simulink model "Aerosonde_NON_linear"  (R2023b)
settings: Solver=VariableStepAuto  StartTime=0.0  StopTime=30  RelTol=1e-3
InitFcn:
  | X0 = [0; 2; -0.25; 0.01; 0; 0; 0; 0; 0; 0; 0; 0]
values from neighbouring files (symbols this model uses):
  kd_pitch = (2*zita_pitch * wn_pitch -a_teta1)/a_teta3    [aerosonde_NON_linear_model.m]
  kd_roll = (2*zita_phi*wn_roll-a_phi1)/a_phi2    [aerosonde_NON_linear_model.m]
  ki_beta = wn_beta^2/a_beta2    (= -1631.35406636)    [aerosonde_NON_linear_model.m]
  ki_course = wn_course^2*Vg/gravity    [aerosonde_NON_linear_model.m]
  ki_h = wn_h^2/(Va*K_pitch_DC)    [aerosonde_NON_linear_model.m]
  ki_v = wn_V^2 / a_v2    (= 0.410281846391)    [aerosonde_NON_linear_model.m]
  ki_v2 = -wn_V2^2/gravity/K_pitch_DC    [aerosonde_NON_linear_model.m]
  kp_beta = delta_r_max/e_beta_max    (= -61)    [aerosonde_NON_linear_model.m]
  kp_course = 2*zita_course*wn_course*Vg/gravity    [aerosonde_NON_linear_model.m]
  kp_h = 2*zita_h*wn_h/(Va*K_pitch_DC)    [aerosonde_NON_linear_model.m]
  kp_pitch = delta_e_max / e_teta_max * sign(a_teta3)    [aerosonde_NON_linear_model.m]
  kp_roll = delta_a_max/e_phi_max    (= 1.04)    [aerosonde_NON_linear_model.m]
  kp_v = (2*zita_V*wn_V-a_v1)/a_v2    (= 0.315424848104)    [aerosonde_NON_linear_model.m]
  kp_v2 = -(a_v1 - 2*zita_V2 * wn_V2)/gravity/K_pitch_DC    [aerosonde_NON_linear_model.m]
  Lu = 300    [aerosonde_NON_linear_model.m]
  Lv = Lu    (= 300)    [aerosonde_NON_linear_model.m]
  Lw = 100    [aerosonde_NON_linear_model.m]
  sigma_u = 2.12    [aerosonde_NON_linear_model.m]
  sigma_v = sigma_u    (= 2.12)    [aerosonde_NON_linear_model.m]
  sigma_w = 1.4    [aerosonde_NON_linear_model.m]
  Va = [0.01 0.01 0.0102487877003 0.0114927261887 0.0177124182161 0.0248890223027 0.0320656246486 0.0395378524425 0.0423652294331 0.0451926059638 0.0466645323698 0.0481364586384 ... (831 elements, 831x1)]    [Vae1.mat]    (also in Vae2.mat = [0.01 0.01 0.0102487877003 0.0114927261887 0.0177124182161 0; Vae3.mat = [0.01 0.01 0.0102487877003 0.0114927261887 0.0177124182161 0; Vze2.mat = [0.01 0.01 0.0102487877003 0.0114927261887 0.0177124182161 0; Vze3.mat = [0.01 0.01 0.0102487877003 0.0114927261887 0.0177124182161 0)
libraries: simulink_extras x15, slpidlib x6, simulink x2, sim3dlib x1, uavsim3dlib x1
settings Model: Creator=Marco  LastModifiedBy=sasi
settings SolverCC: ZeroCrossAlgorithm=Adaptive
settings DebuggingCC: IgnoredZcDiagnostic=none  UnconnectedInputMsg=warning  UnconnectedOutputMsg=warning  UnconnectedLineMsg=warning
settings ModelReferenceCC: EnableRefExpFcnMdlSchedulingChecks=on
settings RTWCC: DLArmComputeVersion=19.05

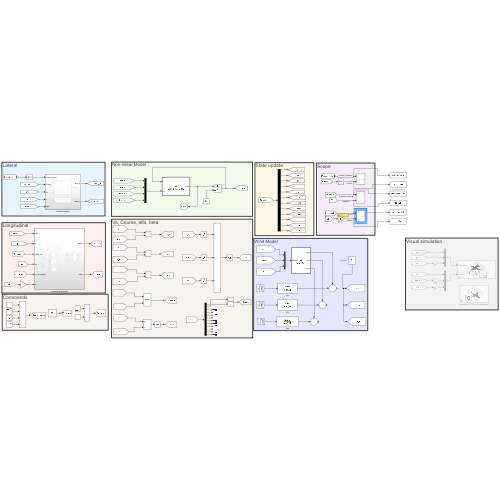
[thumbnail: Simulink's stored preview of the top-level diagram]
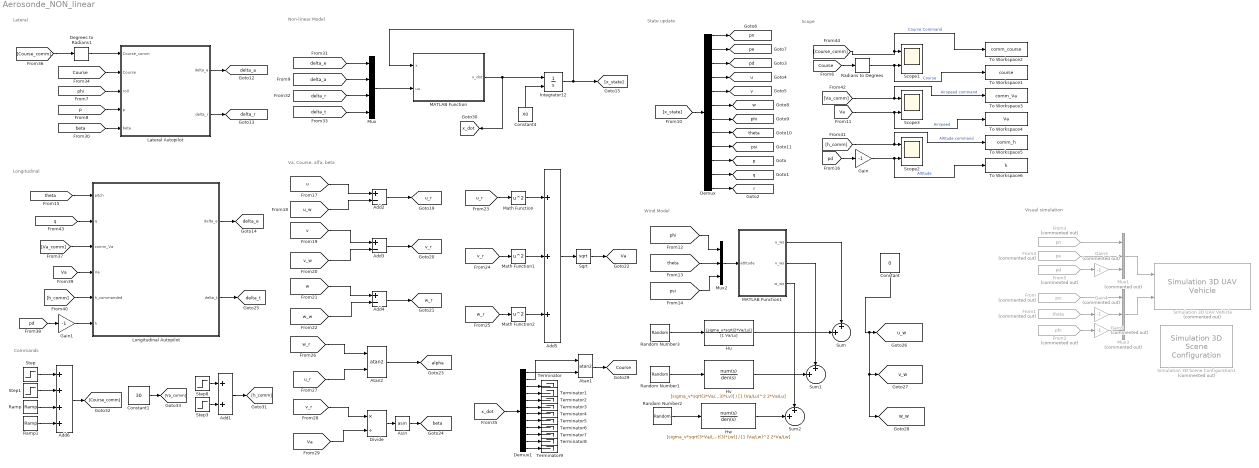
== system Aerosonde_NON_linear ==
  note: Va, Course, alfa, beta
  note: Visual simulation
  note: State update
  note: Scope
  note: Commands
  note: Wind Model
  note: Non-linear Model
  note: Longitudinal
  note: Lateral
  Add1 : Sum
  Add2 : Sum  Inputs=+-
  Add3 : Sum  Inputs=+-
  Add4 : Sum  Inputs=+-
  Add5 : Sum  Inputs=+++
  Add6 : Sum  Inputs=++++
  Asin : Trigonometry  Operator=asin
  Atan1 : Trigonometry  Operator=atan2
  Atan2 : Trigonometry  Operator=atan2
  Constant : Constant  Value=0
  Constant1 : Constant  Value=30
  Constant4 : Constant  Value=X0
  Degrees to Radians1 : simulink_extras/Transformations/Degrees to Radians
  Demux : Demux  Outputs=12
  Demux1 : Demux  Outputs=12
  Divide : Product  Inputs=*/
  From : From  Commented=on  GotoTag=psi  TagVisibility=global
  From1 : From  Commented=on  GotoTag=theta  TagVisibility=global
  From2 : From  Commented=on  GotoTag=phi  TagVisibility=global
  From3 : From  Commented=on  GotoTag=pn  TagVisibility=global
  From4 : From  Commented=on  GotoTag=pe  TagVisibility=global
  From5 : From  Commented=on  GotoTag=pd  TagVisibility=global
  Gain : Gain  Gain=-1
  Gain1 : Gain  Gain=-1
  Gain3 : Gain  Commented=on  Gain=-1
  Gain4 : Gain  Commented=on  Gain=-1
  Gain5 : Gain  Commented=on  Gain=-1
  Hu : TransferFcn  Numerator=[sigma_u*sqrt(2*Va/Lu)]  Denominator=[1 Va/Lu]
  Hv : TransferFcn  Numerator=[sigma_v*sqrt(3*Va/Lu) Va/(sqrt(3)*Lv)]  Denominator=[1 (Va/Lu)^2 2*Va/Lu]
  Hw : TransferFcn  Numerator=[sigma_v*sqrt(3*Va/Lw) Va/(sqrt(3)*Lw)]  Denominator=[1 (Va/Lw)^2 2*Va/Lw]
  Integrator12 : Integrator  InitialConditionSource=external
  Lateral Autopilot : Subsystem
  Longitudinal Autopilot : Subsystem
  MATLAB Function : MATLAB Function  TreatAsAtomicUnit=on
  MATLAB Function1 : MATLAB Function  TreatAsAtomicUnit=on
  Math Function : Math  Operator=square
  Math Function1 : Math  Operator=square
  Math Function2 : Math  Operator=square
  Mux : Mux
  Mux1 : Mux  Commented=on  Inputs=3
  Mux2 : Mux  Inputs=3
  Mux3 : Mux  Commented=on  Inputs=3
  Radians to Degrees : simulink_extras/Transformations/Radians to Degrees
  Ramp : simulink/Sources/Ramp  slope=-tan(deg2rad(85))  start=50  InitialOutput=0
  Ramp1 : simulink/Sources/Ramp  slope=tan(deg2rad(85))  start=60  InitialOutput=0
  Random Number1 : RandomNumber  Variance=sigma_v  SampleTime=0.1
  Random Number2 : RandomNumber  Variance=sigma_w  SampleTime=0.1
  Random Number3 : RandomNumber  Variance=sigma_u  SampleTime=0.1
  Scope1 : Scope  NumInputPorts=2
  Scope2 : Scope  NumInputPorts=2
  Scope3 : Scope  NumInputPorts=2
  Simulation 3D Scene Configuration1 : sim3dlib/Simulation 3D Scene Configuration  Priority=0  Commented=on  ProjectFormat=Default Scenes  SceneDesc=Airport  ProjectName=C:\Program Files\MATLAB\R2023b\toolbox\shared\sim3d_projects\automotive_project_windows\UE\WindowsNoEditor\VehicleSimulation.exe  ScenePath=/Game/Maps/HwStrght  EnableOpenDRIVE=off  vehTagList={'Scene Origin';'SimulinkVehicle1'}  vehTag=SimulinkVehicle1  FreeCameraInitialTranslation=[0, 0, 0]  FreeCameraDefaultInitialTranslation=[-6, 0, 2]  FreeCameraInitialRotation=[0, 0, 0]  FreeCameraDefaultInitialRotation=[0, -15, 0]  OpVisEn=off  Ts=.02  EnableWindow=on  EnableRemoteAccess=off  EnableWeather=off  SunAltitude=40.0  SunAzimuth=90  clouds=10  wind=1  fog=0  rain=0  EnableGeospatial=off  OriginHeight=200  OriginLatitude=40.744652  OriginLongitude=-73.988864  MapStyle=Aerial  AdditionalAssetIDs=[]  UseAdvancedSunSky=off  SolarTime=11  TimeZone=-5  Day=21  Month=9  Year=2022  UseDaylightSavingTime=on  DSTStartDay=10  DSTStartMonth=3  DSTEndDay=3  DSTEndMonth=11  DSTSwitchHour=2  sensorTag=MainCamera2  sensorId=2  sensorName=MainCamera2  mountLoc=Origin  offsetFlag=off  tmountOffset=[0, 0, 0]  rmountOffset=[0, 0, 0]  HorizontalResolution=1280  VerticalResolution=720  HorizontalFOV=60  mountPoint=[0 0 0]  mountOrientation=[0 0 0]  aMode=0  ID=2  GeoTrigger=Inactive
      settings: LibrarySourceBlock=aerolibsim3d/Simulation 3D Scene Configuration
  Simulation 3D UAV Vehicle : uavsim3dlib/Simulation 3D UAV Vehicle  Priority=-1  Commented=on  Mesh=Fixed wing  MeshPath=/MathWorksUAVContent/UAVs/HexaRotorUAV/HexaRotor.HexaRotor  Color=Red  ActorName=SimulinkVehicle1  UseGlobalFrame=off  InitialTranslation=[0 0 0]  InitialRotation=[0 0 0]  InitialTranslationGlobal=[0 0 0]  InitialGeoOrigin=[0 0 0]  InitialRotationGlobal=[0 0 0]  SampleTime=-1  ActorType=SimulinkVehicle  ID=1  aMode=4  ActorTag=SimulinkVehicle1
  Sqrt : Sqrt
  Step : Step  Time=31  After=40  SampleTime=0
  Step1 : Step  Time=39  After=-80  SampleTime=0
  Step3 : Step  Time=15  After=-60  SampleTime=0
  Step8 : Step  Time=0  After=120  SampleTime=0
  Sum : Sum  Inputs=++|
  Sum1 : Sum  Inputs=++|
  Sum2 : Sum  Inputs=++|
  Terminator{,1..9} (10 alike) : Terminator
  To Workspace1 : ToWorkspace  VariableName=course  SampleTime=-1
      settings: Save2DSignal=2-D array (concatenate along first dimension)
  To Workspace2 : ToWorkspace  VariableName=comm_course  SampleTime=-1
      settings: Save2DSignal=2-D array (concatenate along first dimension)
  To Workspace3 : ToWorkspace  VariableName=comm_Va  SampleTime=-1
      settings: Save2DSignal=2-D array (concatenate along first dimension)
  To Workspace4 : ToWorkspace  VariableName=Va  SampleTime=-1
      settings: Save2DSignal=2-D array (concatenate along first dimension)
  To Workspace5 : ToWorkspace  VariableName=comm_h  SampleTime=-1
      settings: Save2DSignal=2-D array (concatenate along first dimension)
  To Workspace6 : ToWorkspace  VariableName=h  SampleTime=-1
      settings: Save2DSignal=2-D array (concatenate along first dimension)
  tag scope: Course=global, Va=global, alpha=global, beta=global, delta_a=global, delta_e=global, delta_r=global, delta_t=global, p=global, pd=global, pe=global, phi=global, pn=global, psi=global, q=global, r=global, theta=global, u=global, u_r=global, u_w=global, v=global, v_r=global, v_w=global, w=global, w_r=global, w_w=global, x_dot=global
  wires:
  MATLAB Function/1(x_dot) -> Integrator12/1, [x_dot]
  Mux/1 -> MATLAB Function/2(uu)
  Integrator12/1 -> MATLAB Function/1(x), [x_state]
  Constant4/1 -> Integrator12/2
  Mux1/1 -> Simulation 3D UAV Vehicle/1
  Mux3/1 -> Simulation 3D UAV Vehicle/2
  Demux/10 -> [p]
  Demux/11 -> [q]
  Demux/12 -> [r]
  Demux/9 -> [psi]
  Demux/8 -> [theta]
  Demux/6 -> [w]
  Demux/7 -> [phi]
  Demux/5 -> [v]
  Demux/4 -> [u]
  Demux/3 -> [pd]
  Demux/2 -> [pe]
  Demux/1 -> [pn]
  From/1 -> Mux3/1
  From4/1 -> Mux1/2
  From3/1 -> Mux1/1
  Degrees to Radians1/1 -> Lateral Autopilot/1(Course_comm)
  [u] -> Add2/1
  [w] -> Add4/1
  [w_w] -> Add4/2
  [v] -> Add3/1
  [v_w] -> Add3/2
  [u_w] -> Add2/2
  Add2/1 -> [u_r]
  Add3/1 -> [v_r]
  Add4/1 -> [w_r]
  [u_r] -> Math Function/1
  [v_r] -> Math Function1/1
  [w_r] -> Math Function2/1
  Math Function2/1 -> Add5/3
  Math Function1/1 -> Add5/2
  Math Function/1 -> Add5/1
  Add5/1 -> Sqrt/1
  Sqrt/1 -> [Va]
  [w_r] -> Atan2/1
  [u_r] -> Atan2/2
  Atan2/1 -> [alpha]
  [v_r] -> Divide/1
  [Va] -> Divide/2
  Divide/1 -> Asin/1
  Asin/1 -> [beta]
  [delta_e] -> Mux/1
  From5/1 -> Gain3/1
  Gain3/1 -> Mux1/3
  From1/1 -> Gain4/1
  Gain4/1 -> Mux3/2
  From2/1 -> Gain5/1
  Gain5/1 -> Mux3/3
  [delta_a] -> Mux/2
  [delta_r] -> Mux/3
  [delta_t] -> Mux/4
  [x_state] -> Demux/1
  Mux2/1 -> MATLAB Function1/1(attitude)
  [theta] -> Mux2/2
  [phi] -> Mux2/1
  [psi] -> Mux2/3
  MATLAB Function1/1(u_ws) -> Sum/1
  MATLAB Function1/2(v_ws) -> Sum1/1
  MATLAB Function1/3(w_ws) -> Sum2/1
  [phi] -> Lateral Autopilot/3(roll)
  [p] -> Lateral Autopilot/4(p)
  [beta] -> Lateral Autopilot/5(beta)
  Lateral Autopilot/1(delta_a) -> [delta_a]
  Lateral Autopilot/2(delta_r) -> [delta_r]
  Demux1/2 -> Atan1/1
  Demux1/1 -> Atan1/2
  [Course] -> Lateral Autopilot/2(Course)
  [x_dot] -> Demux1/1
  Demux1/3 -> Terminator/1
  Demux1/4 -> Terminator1/1
  Demux1/5 -> Terminator2/1
  Demux1/6 -> Terminator3/1
  Demux1/7 -> Terminator4/1
  Demux1/8 -> Terminator5/1
  Demux1/9 -> Terminator6/1
  Demux1/10 -> Terminator7/1
  Demux1/11 -> Terminator8/1
  Demux1/12 -> Terminator9/1
  [pd] -> Gain1/1
  Longitudinal Autopilot/1(delta_e) -> [delta_e]
  [theta] -> Longitudinal Autopilot/1(pitch)
  [q] -> Longitudinal Autopilot/2(q)
  [Va] -> Longitudinal Autopilot/4(Va)
  Gain1/1 -> Longitudinal Autopilot/6(h)
  Longitudinal Autopilot/2(delta_t) -> [delta_t]
  Atan1/1 -> [Course]
  [pd] -> Gain/1
  [Course_comm] -> Degrees to Radians1/1
  [Va_comm] -> Longitudinal Autopilot/3(comm_Va)
  [h_comm] -> Longitudinal Autopilot/5(h_commanded)
  [Course_comm] -> To Workspace2/1, Scope1/1  "Course Command"
  [Course] -> Radians to Degrees/1
  [Va_comm] -> To Workspace3/1, Scope3/1  "Airspeed command"
  [Va] -> To Workspace4/1, Scope3/2  "Airspeed"
  [h_comm] -> To Workspace5/1, Scope2/1  "Altitude command"
  Gain/1 -> To Workspace6/1, Scope2/2  "Altitude"
  Radians to Degrees/1 -> To Workspace1/1, Scope1/2  "Course"
  Constant1/1 -> [Va_comm]
  Step8/1 -> Add1/1
  Add1/1 -> [h_comm]
  Step/1 -> Add6/1
  Step1/1 -> Add6/2
  Ramp/1 -> Add6/3
  Ramp1/1 -> Add6/4
  Step3/1 -> Add1/2
  Add6/1 -> [Course_comm]
  Hw/1 -> Sum2/2
  Hv/1 -> Sum1/2
  Random Number3/1 -> Hu/1
  Hu/1 -> Sum/2
  Random Number1/1 -> Hv/1
  Random Number2/1 -> Hw/1
  Constant/1 -> [w_w], [v_w], [u_w]

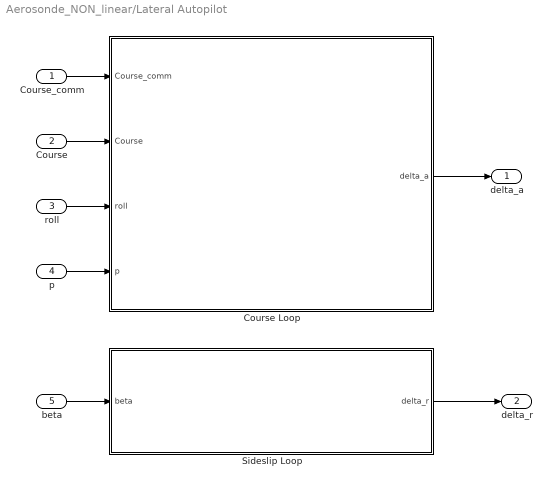
== system Aerosonde_NON_linear/Lateral Autopilot ==
  Course_comm : Inport
  Course : Inport  Port=2
  roll : Inport  Port=3
  p : Inport  Port=4
  beta : Inport  Port=5
  Course Loop : Subsystem
  Sideslip Loop : Subsystem
  delta_a : Outport
  delta_r : Outport  Port=2
  wires:
  beta/1 -> Sideslip Loop/1(beta)
  p/1 -> Course Loop/4(p)
  Course Loop/1(delta_a) -> delta_a/1
  Course_comm/1 -> Course Loop/1(Course_comm)
  Sideslip Loop/1(delta_r) -> delta_r/1
  roll/1 -> Course Loop/3(roll)
  Course/1 -> Course Loop/2(Course)

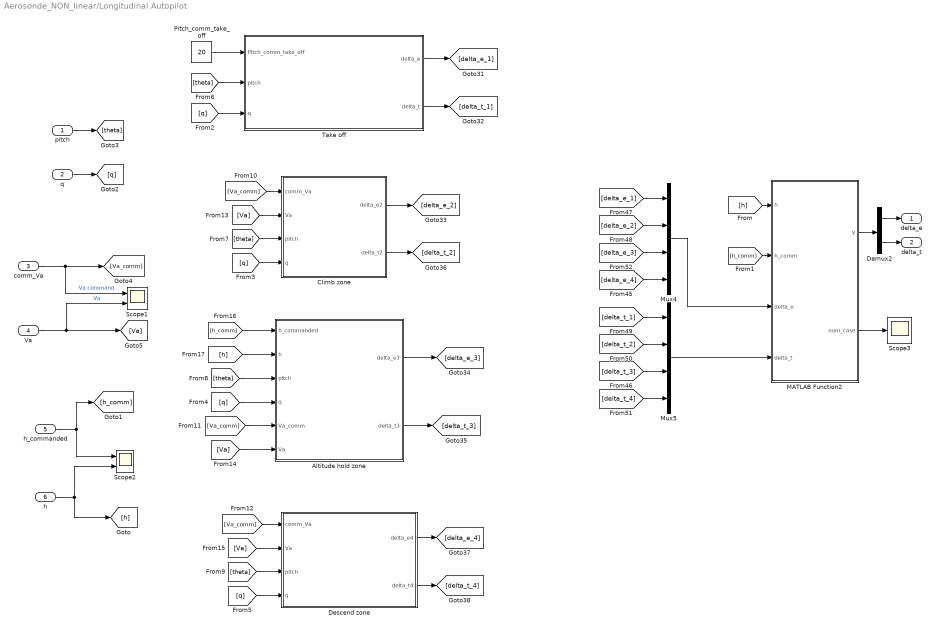
== system Aerosonde_NON_linear/Longitudinal Autopilot ==
  pitch : Inport
  q : Inport  Port=2
  comm_Va : Inport  Port=3
  Va : Inport  Port=4
  h_commanded : Inport  Port=5
  h : Inport  Port=6
  Altitude hold zone : Subsystem
  Climb zone : Subsystem
  Demux2 : Demux  Outputs=2
  Descend zone : Subsystem
  MATLAB Function2 : MATLAB Function  TreatAsAtomicUnit=on
  Mux4 : Mux
  Mux5 : Mux
  Pitch_comm_take_off : Constant  Value=20
  Scope1 : Scope  NumInputPorts=2
  Scope2 : Scope  NumInputPorts=2
  Scope3 : Scope
  Take off : Subsystem  TreatAsAtomicUnit=on
  delta_e : Outport
  delta_t : Outport  Port=2
  wires:
  [delta_t_1] -> Mux5/1
  Demux2/2 -> delta_t/1
  Descend zone/1(delta_e4) -> [delta_e_4]
  Mux5/1 -> MATLAB Function2/4(delta_t)
  h/1 -> Scope2/2, [h]
  Demux2/1 -> delta_e/1
  [delta_e_2] -> Mux4/2
  [delta_e_4] -> Mux4/4
  [delta_t_3] -> Mux5/3
  MATLAB Function2/2(num_case) -> Scope3/1
  Climb zone/1(delta_e2) -> [delta_e_2]
  [delta_t_2] -> Mux5/2
  [delta_e_3] -> Mux4/3
  [delta_t_4] -> Mux5/4
  Mux4/1 -> MATLAB Function2/3(delta_e)
  [delta_e_1] -> Mux4/1
  Descend zone/2(delta_t4) -> [delta_t_4]
  Take off/1(delta_e) -> [delta_e_1]
  Climb zone/2(delta_t2) -> [delta_t_2]
  Take off/2(delta_t) -> [delta_t_1]
  Altitude hold zone/2(delta_t3) -> [delta_t_3]
  Altitude hold zone/1(delta_e3) -> [delta_e_3]
  MATLAB Function2/1(y) -> Demux2/1
  h_commanded/1 -> Scope2/1, [h_comm]
  Pitch_comm_take_off/1 -> Take off/1(Pitch_comm_take_off)
  comm_Va/1 -> Scope1/1, [Va_comm]  "Va command"
  Va/1 -> Scope1/2, [Va]  "Va"
  pitch/1 -> [theta]
  [h] -> MATLAB Function2/1(h)
  [h_comm] -> MATLAB Function2/2(h_comm)
  [q] -> Take off/3(q)
  [q] -> Climb zone/4(q)
  [q] -> Altitude hold zone/4(q)
  [q] -> Descend zone/4(q)
  q/1 -> [q]
  [theta] -> Take off/2(pitch)
  [theta] -> Climb zone/3(pitch)
  [theta] -> Altitude hold zone/3(pitch)
  [theta] -> Descend zone/3(pitch)
  [Va_comm] -> Climb zone/1(comm_Va)
  [Va_comm] -> Altitude hold zone/5(Va_comm)
  [Va_comm] -> Descend zone/1(comm_Va)
  [Va] -> Climb zone/2(Va)
  [Va] -> Altitude hold zone/6(Va)
  [Va] -> Descend zone/2(Va)
  [h_comm] -> Altitude hold zone/1(h_commanded)
  [h] -> Altitude hold zone/2(h)

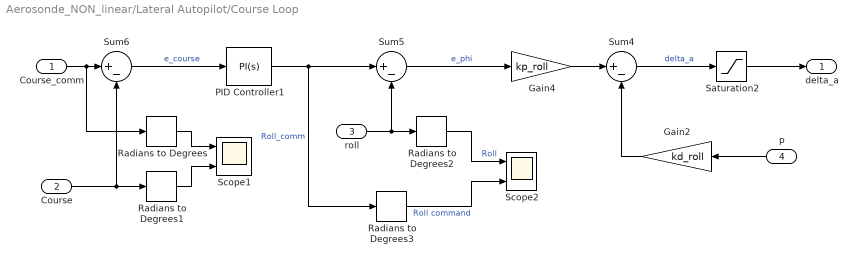
== system Aerosonde_NON_linear/Lateral Autopilot/Course Loop ==
  Course_comm : Inport
  Course : Inport  Port=2
  roll : Inport  Port=3
  p : Inport  Port=4
  Gain2 : Gain  Gain=kd_roll
  Gain4 : Gain  Gain=kp_roll
  PID Controller1 : slpidlib/PID Controller  Controller=PI  Form=Parallel  TimeDomain=Continuous-time  UseExternalTs=off  SampleTime=-1  IntegratorMethod=Forward Euler  FilterMethod=Forward Euler  ControllerParametersSource=internal  P=kp_course  I=ki_course  UseKiTs=off  D=0  N=100  UseFilter=on  TunerSelectOption=Transfer Function Based (PID Tuner App)  InitialConditionSource=internal  InitialConditionForIntegrator=0  InitialConditionForFilter=0  DifferentiatorICPrevScaledInput=0  ExternalReset=none  TrackingMode=off  Kt=1  LimitOutput=on  SatLimitsSource=internal  UpperSaturationLimit=deg2rad(40)  LowerSaturationLimit=deg2rad(-40)  LinearizeAsGain=on  AntiWindupMode=clamping  Kb=1  LimitIntegrator=off  UpperIntegratorSaturationLimit=inf  LowerIntegratorSaturationLimit=-inf  POutMin=[]  POutMax=[]  IOutMin=[]  IOutMax=[]  DOutMin=[]  DOutMax=[]  NOutMin=[]  NOutMax=[]  SumOutMin=[]  SumOutMax=[]  SaturationOutMin=[]  SaturationOutMax=[]  PParamMin=[]  PParamMax=[]  IParamMin=[]  IParamMax=[]  DParamMin=[]  DParamMax=[]  NParamMin=[]  NParamMax=[]  KbParamMin=[]  KbParamMax=[]  KtParamMin=[]  KtParamMax=[]  KbOutMin=[]  KbOutMax=[]  KtOutMin=[]  KtOutMax=[]  IntegratorOutMin=[]  IntegratorOutMax=[]  FilterOutMin=[]  FilterOutMax=[]  SumI1OutMin=[]  SumI1OutMax=[]  SumI2OutMin=[]  SumI2OutMax=[]  SumI3OutMin=[]  SumI3OutMax=[]  SumI4OutMin=[]  SumI4OutMax=[]  SumDOutMin=[]  SumDOutMax=[]  DifferentiatorOutMin=[]  DifferentiatorOutMax=[]  FilterDiffOutCoefMin=[]  FilterDiffOutCoefMax=[]  ReciprocalOutMin=[]  ReciprocalOutMax=[]  SumDenOutMin=[]  SumDenOutMax=[]  SumNumOutMin=[]  SumNumOutMax=[]  DivideOutMin=[]  DivideOutMax=[]  UdiffTsProdOutMin=[]  UdiffTsProdOutMax=[]  NTsProdOutMin=[]  NTsProdOutMax=[]  UintegralTsProdOutMin=[]  UintegralTsProdOutMax=[]  UngainTsProdOutMin=[]  UngainTsProdOutMax=[]  ClampingZeroOutDataTypeStr=Inherit: Inherit via back propagation  ClampingZeroOutMin=[]  ClampingZeroOutMax=[]  FilterDenConstantOutDataTypeStr=Inherit: Inherit via back propagation  FilterDenConstantOutMin=[]  FilterDenConstantOutMax=[]  PCopyOutDataTypeStr=Inherit: Inherit via back propagation  PCopyOutMin=[]  PCopyOutMax=[]  NCopyOutDataTypeStr=Inherit: Inherit via back propagation  NCopyOutMin=[]  NCopyOutMax=[]  IntegratorContinuousStateAttributes=''  IntegratorStateMustResolveToSignalObject=off  IntegratorRTWStateStorageClass=Auto  FilterContinuousStateAttributes=''  FilterStateMustResolveToSignalObject=off  FilterRTWStateStorageClass=Auto  ParallelPVariant=InternalParameters  IdealPVariant=Disabled  IVariant=InternalParameters  DVariant=Disabled  IntegratorVariant=Continuous  SatVariant=Enabled  AWVariant=ContClampingParallel  PCopyVariant=Disabled  TRVariant=Disabled  FdbkBlocksVariant=Forward  IdealPFdbkVariant=Disabled  SatFdbkVariant=Disabled  DerivativeFilterVariant=Disabled  NVariant=Disabled  NCopyVariant=Disabled_SignalSpec  FilterICVariant=Disabled  IntegratorICVariant=InternalICs  ExternalResetVariant=Disabled  TRSumVariant=Passthrough  SumFdbkVariant=Disabled  SumVariant=Sum_PI  TsampFilterVariant=InternalTs  TsampNgainVariant=Passthrough  TsampIntegralVariant=Disabled_SignalSpec  ExternalSaturationOutDataTypeStr=Inherit: Same as second input
  Radians to Degrees{,1..3} (4 alike) : simulink_extras/Transformations/Radians to Degrees
  Saturation2 : Saturate  UpperLimit=0.52  LowerLimit=-0.52
  Scope1 : Scope  NumInputPorts=2
  Scope2 : Scope  NumInputPorts=2
  Sum4 : Sum  Inputs=|+-
  Sum5 : Sum  Inputs=|+-
  Sum6 : Sum  Inputs=|+-
  delta_a : Outport
  wires:
  Course_comm/1 -> Radians to Degrees/1, Sum6/1
  Sum6/1 -> PID Controller1/1  "e_course"
  Sum4/1 -> Saturation2/1  "delta_a"
  Gain4/1 -> Sum4/1
  Gain2/1 -> Sum4/2
  Sum5/1 -> Gain4/1  "e_phi"
  Saturation2/1 -> delta_a/1
  roll/1 -> Radians to Degrees2/1, Sum5/2
  p/1 -> Gain2/1
  Course/1 -> Sum6/2, Radians to Degrees1/1
  PID Controller1/1 -> Sum5/1, Radians to Degrees3/1  "Roll_comm"
  Radians to Degrees/1 -> Scope1/1
  Radians to Degrees1/1 -> Scope1/2
  Radians to Degrees2/1 -> Scope2/1  "Roll"
  Radians to Degrees3/1 -> Scope2/2  "Roll command"

== system Aerosonde_NON_linear/Lateral Autopilot/Sideslip Loop ==
  beta : Inport
  PID Controller4 : slpidlib/PID Controller  Controller=PI  Form=Parallel  TimeDomain=Continuous-time  UseExternalTs=off  SampleTime=-1  IntegratorMethod=Forward Euler  FilterMethod=Forward Euler  ControllerParametersSource=internal  P=kp_beta  I=ki_beta  UseKiTs=off  D=0  N=100  UseFilter=on  TunerSelectOption=Transfer Function Based (PID Tuner App)  InitialConditionSource=internal  InitialConditionForIntegrator=0  InitialConditionForFilter=0  DifferentiatorICPrevScaledInput=0  ExternalReset=none  TrackingMode=off  Kt=1  LimitOutput=on  SatLimitsSource=internal  UpperSaturationLimit=0.61  LowerSaturationLimit=-0.61  LinearizeAsGain=on  AntiWindupMode=clamping  Kb=1  LimitIntegrator=off  UpperIntegratorSaturationLimit=inf  LowerIntegratorSaturationLimit=-inf  POutMin=[]  POutMax=[]  IOutMin=[]  IOutMax=[]  DOutMin=[]  DOutMax=[]  NOutMin=[]  NOutMax=[]  SumOutMin=[]  SumOutMax=[]  SaturationOutMin=[]  SaturationOutMax=[]  PParamMin=[]  PParamMax=[]  IParamMin=[]  IParamMax=[]  DParamMin=[]  DParamMax=[]  NParamMin=[]  NParamMax=[]  KbParamMin=[]  KbParamMax=[]  KtParamMin=[]  KtParamMax=[]  KbOutMin=[]  KbOutMax=[]  KtOutMin=[]  KtOutMax=[]  IntegratorOutMin=[]  IntegratorOutMax=[]  FilterOutMin=[]  FilterOutMax=[]  SumI1OutMin=[]  SumI1OutMax=[]  SumI2OutMin=[]  SumI2OutMax=[]  SumI3OutMin=[]  SumI3OutMax=[]  SumI4OutMin=[]  SumI4OutMax=[]  SumDOutMin=[]  SumDOutMax=[]  DifferentiatorOutMin=[]  DifferentiatorOutMax=[]  FilterDiffOutCoefMin=[]  FilterDiffOutCoefMax=[]  ReciprocalOutMin=[]  ReciprocalOutMax=[]  SumDenOutMin=[]  SumDenOutMax=[]  SumNumOutMin=[]  SumNumOutMax=[]  DivideOutMin=[]  DivideOutMax=[]  UdiffTsProdOutMin=[]  UdiffTsProdOutMax=[]  NTsProdOutMin=[]  NTsProdOutMax=[]  UintegralTsProdOutMin=[]  UintegralTsProdOutMax=[]  UngainTsProdOutMin=[]  UngainTsProdOutMax=[]  ClampingZeroOutDataTypeStr=Inherit: Inherit via back propagation  ClampingZeroOutMin=[]  ClampingZeroOutMax=[]  FilterDenConstantOutDataTypeStr=Inherit: Inherit via back propagation  FilterDenConstantOutMin=[]  FilterDenConstantOutMax=[]  PCopyOutDataTypeStr=Inherit: Inherit via back propagation  PCopyOutMin=[]  PCopyOutMax=[]  NCopyOutDataTypeStr=Inherit: Inherit via back propagation  NCopyOutMin=[]  NCopyOutMax=[]  IntegratorContinuousStateAttributes=''  IntegratorStateMustResolveToSignalObject=off  IntegratorRTWStateStorageClass=Auto  FilterContinuousStateAttributes=''  FilterStateMustResolveToSignalObject=off  FilterRTWStateStorageClass=Auto  ParallelPVariant=InternalParameters  IdealPVariant=Disabled  IVariant=InternalParameters  DVariant=Disabled  IntegratorVariant=Continuous  SatVariant=Enabled  AWVariant=ContClampingParallel  PCopyVariant=Disabled  TRVariant=Disabled  FdbkBlocksVariant=Forward  IdealPFdbkVariant=Disabled  SatFdbkVariant=Disabled  DerivativeFilterVariant=Disabled  NVariant=Disabled  NCopyVariant=Disabled_SignalSpec  FilterICVariant=Disabled  IntegratorICVariant=InternalICs  ExternalResetVariant=Disabled  TRSumVariant=Passthrough  SumFdbkVariant=Disabled  SumVariant=Sum_PI  TsampFilterVariant=InternalTs  TsampNgainVariant=Passthrough  TsampIntegralVariant=Disabled_SignalSpec  ExternalSaturationOutDataTypeStr=Inherit: Same as second input
  Radians to Degrees : simulink_extras/Transformations/Radians to Degrees
  Scope2 : Scope
  delta_r : Outport
  wires:
  beta/1 -> Radians to Degrees/1, PID Controller4/1  "e_beta"
  PID Controller4/1 -> delta_r/1  "delta_r"
  Radians to Degrees/1 -> Scope2/1  "Beta"

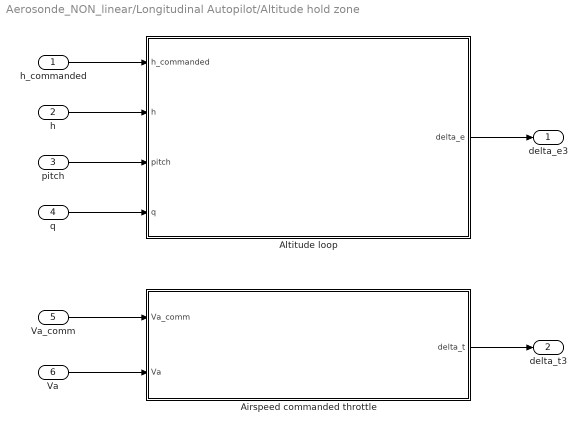
== system Aerosonde_NON_linear/Longitudinal Autopilot/Altitude hold zone ==
  h_commanded : Inport
  h : Inport  Port=2
  pitch : Inport  Port=3
  q : Inport  Port=4
  Va_comm : Inport  Port=5
  Va : Inport  Port=6
  Airspeed commanded throttle : Subsystem
  Altitude loop : Subsystem
  delta_e3 : Outport
  delta_t3 : Outport  Port=2
  wires:
  Airspeed commanded throttle/1(delta_t) -> delta_t3/1
  Va_comm/1 -> Airspeed commanded throttle/1(Va_comm)
  Va/1 -> Airspeed commanded throttle/2(Va)
  q/1 -> Altitude loop/4(q)
  h/1 -> Altitude loop/2(h)
  pitch/1 -> Altitude loop/3(pitch)
  h_commanded/1 -> Altitude loop/1(h_commanded)
  Altitude loop/1(delta_e) -> delta_e3/1

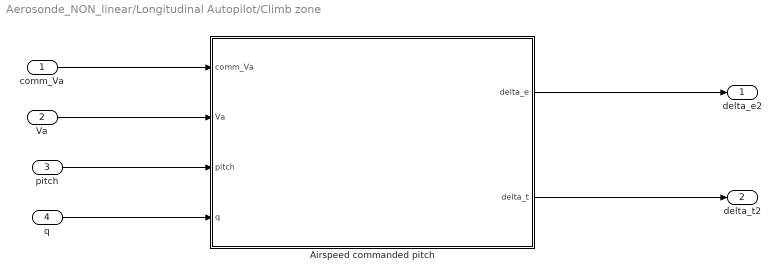
== system Aerosonde_NON_linear/Longitudinal Autopilot/Climb zone ==
  comm_Va : Inport
  Va : Inport  Port=2
  pitch : Inport  Port=3
  q : Inport  Port=4
  Airspeed commanded pitch : Subsystem
  delta_e2 : Outport
  delta_t2 : Outport  Port=2
  wires:
  comm_Va/1 -> Airspeed commanded pitch/1(comm_Va)
  Airspeed commanded pitch/1(delta_e) -> delta_e2/1
  Va/1 -> Airspeed commanded pitch/2(Va)
  q/1 -> Airspeed commanded pitch/4(q)
  Airspeed commanded pitch/2(delta_t) -> delta_t2/1
  pitch/1 -> Airspeed commanded pitch/3(pitch)

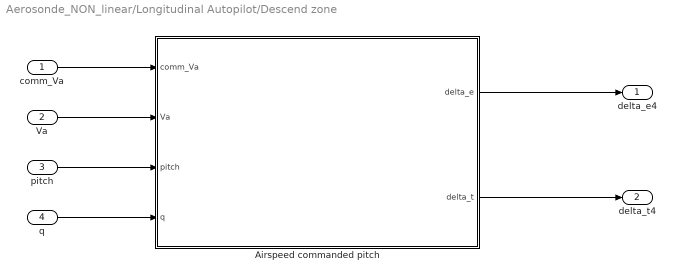
== system Aerosonde_NON_linear/Longitudinal Autopilot/Descend zone ==
  comm_Va : Inport
  Va : Inport  Port=2
  pitch : Inport  Port=3
  q : Inport  Port=4
  Airspeed commanded pitch : Subsystem
  delta_e4 : Outport
  delta_t4 : Outport  Port=2
  wires:
  comm_Va/1 -> Airspeed commanded pitch/1(comm_Va)
  Airspeed commanded pitch/1(delta_e) -> delta_e4/1
  Va/1 -> Airspeed commanded pitch/2(Va)
  q/1 -> Airspeed commanded pitch/4(q)
  Airspeed commanded pitch/2(delta_t) -> delta_t4/1
  pitch/1 -> Airspeed commanded pitch/3(pitch)

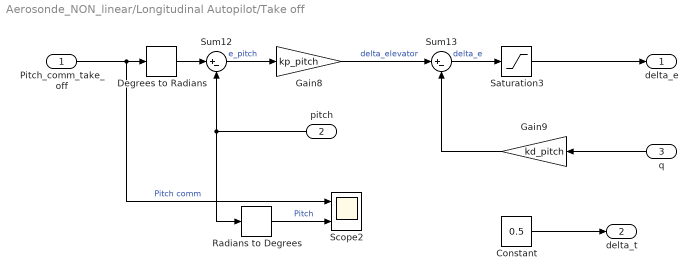
== system Aerosonde_NON_linear/Longitudinal Autopilot/Take off ==
  Pitch_comm_take_off : Inport
  pitch : Inport  Port=2
  q : Inport  Port=3
  Constant : Constant  Value=0.5
  Degrees to Radians : simulink_extras/Transformations/Degrees to Radians
  Gain8 : Gain  Gain=kp_pitch
  Gain9 : Gain  Gain=kd_pitch
  Radians to Degrees : simulink_extras/Transformations/Radians to Degrees
  Saturation3 : Saturate  UpperLimit=0.43  LowerLimit=-0.43
  Scope2 : Scope  NumInputPorts=2
  Sum12 : Sum  Inputs=|+-
  Sum13 : Sum  Inputs=|+-
  delta_e : Outport
  delta_t : Outport  Port=2
  wires:
  Sum13/1 -> Saturation3/1  "delta_e"
  Gain9/1 -> Sum13/2
  q/1 -> Gain9/1
  Gain8/1 -> Sum13/1  "delta_elevator"
  Saturation3/1 -> delta_e/1
  pitch/1 -> Sum12/2, Radians to Degrees/1
  Sum12/1 -> Gain8/1  "e_pitch"
  Degrees to Radians/1 -> Sum12/1
  Constant/1 -> delta_t/1
  Pitch_comm_take_off/1 -> Scope2/1, Degrees to Radians/1  "Pitch comm"
  Radians to Degrees/1 -> Scope2/2  "Pitch"

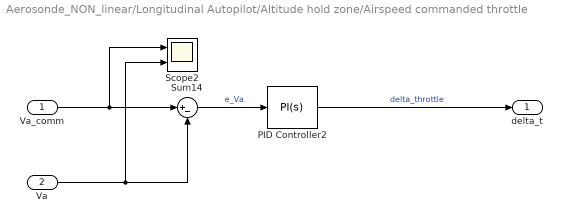
== system Aerosonde_NON_linear/Longitudinal Autopilot/Altitude hold zone/Airspeed commanded throttle ==
  Va_comm : Inport
  Va : Inport  Port=2
  PID Controller2 : slpidlib/PID Controller  Controller=PI  Form=Parallel  TimeDomain=Continuous-time  UseExternalTs=off  SampleTime=-1  IntegratorMethod=Forward Euler  FilterMethod=Forward Euler  ControllerParametersSource=internal  P=kp_v  I=ki_v  UseKiTs=off  D=0  N=100  UseFilter=on  TunerSelectOption=Transfer Function Based (PID Tuner App)  InitialConditionSource=internal  InitialConditionForIntegrator=0  InitialConditionForFilter=0  DifferentiatorICPrevScaledInput=0  ExternalReset=none  TrackingMode=off  Kt=1  LimitOutput=on  SatLimitsSource=internal  UpperSaturationLimit=1  LowerSaturationLimit=0  LinearizeAsGain=on  AntiWindupMode=clamping  Kb=1  LimitIntegrator=off  UpperIntegratorSaturationLimit=inf  LowerIntegratorSaturationLimit=-inf  POutMin=[]  POutMax=[]  IOutMin=[]  IOutMax=[]  DOutMin=[]  DOutMax=[]  NOutMin=[]  NOutMax=[]  SumOutMin=[]  SumOutMax=[]  SaturationOutMin=[]  SaturationOutMax=[]  PParamMin=[]  PParamMax=[]  IParamMin=[]  IParamMax=[]  DParamMin=[]  DParamMax=[]  NParamMin=[]  NParamMax=[]  KbParamMin=[]  KbParamMax=[]  KtParamMin=[]  KtParamMax=[]  KbOutMin=[]  KbOutMax=[]  KtOutMin=[]  KtOutMax=[]  IntegratorOutMin=[]  IntegratorOutMax=[]  FilterOutMin=[]  FilterOutMax=[]  SumI1OutMin=[]  SumI1OutMax=[]  SumI2OutMin=[]  SumI2OutMax=[]  SumI3OutMin=[]  SumI3OutMax=[]  SumI4OutMin=[]  SumI4OutMax=[]  SumDOutMin=[]  SumDOutMax=[]  DifferentiatorOutMin=[]  DifferentiatorOutMax=[]  FilterDiffOutCoefMin=[]  FilterDiffOutCoefMax=[]  ReciprocalOutMin=[]  ReciprocalOutMax=[]  SumDenOutMin=[]  SumDenOutMax=[]  SumNumOutMin=[]  SumNumOutMax=[]  DivideOutMin=[]  DivideOutMax=[]  UdiffTsProdOutMin=[]  UdiffTsProdOutMax=[]  NTsProdOutMin=[]  NTsProdOutMax=[]  UintegralTsProdOutMin=[]  UintegralTsProdOutMax=[]  UngainTsProdOutMin=[]  UngainTsProdOutMax=[]  ClampingZeroOutDataTypeStr=Inherit: Inherit via back propagation  ClampingZeroOutMin=[]  ClampingZeroOutMax=[]  FilterDenConstantOutDataTypeStr=Inherit: Inherit via back propagation  FilterDenConstantOutMin=[]  FilterDenConstantOutMax=[]  PCopyOutDataTypeStr=Inherit: Inherit via back propagation  PCopyOutMin=[]  PCopyOutMax=[]  NCopyOutDataTypeStr=Inherit: Inherit via back propagation  NCopyOutMin=[]  NCopyOutMax=[]  IntegratorContinuousStateAttributes=''  IntegratorStateMustResolveToSignalObject=off  IntegratorRTWStateStorageClass=Auto  FilterContinuousStateAttributes=''  FilterStateMustResolveToSignalObject=off  FilterRTWStateStorageClass=Auto  ParallelPVariant=InternalParameters  IdealPVariant=Disabled  IVariant=InternalParameters  DVariant=Disabled  IntegratorVariant=Continuous  SatVariant=Enabled  AWVariant=ContClampingParallel  PCopyVariant=Disabled  TRVariant=Disabled  FdbkBlocksVariant=Forward  IdealPFdbkVariant=Disabled  SatFdbkVariant=Disabled  DerivativeFilterVariant=Disabled  NVariant=Disabled  NCopyVariant=Disabled_SignalSpec  FilterICVariant=Disabled  IntegratorICVariant=InternalICs  ExternalResetVariant=Disabled  TRSumVariant=Passthrough  SumFdbkVariant=Disabled  SumVariant=Sum_PI  TsampFilterVariant=InternalTs  TsampNgainVariant=Passthrough  TsampIntegralVariant=Disabled_SignalSpec  ExternalSaturationOutDataTypeStr=Inherit: Same as second input
  Scope2 : Scope  NumInputPorts=2
  Sum14 : Sum  Inputs=|+-
  delta_t : Outport
  wires:
  Sum14/1 -> PID Controller2/1  "e_Va"
  Va_comm/1 -> Scope2/1, Sum14/1
  PID Controller2/1 -> delta_t/1  "delta_throttle"
  Va/1 -> Scope2/2, Sum14/2

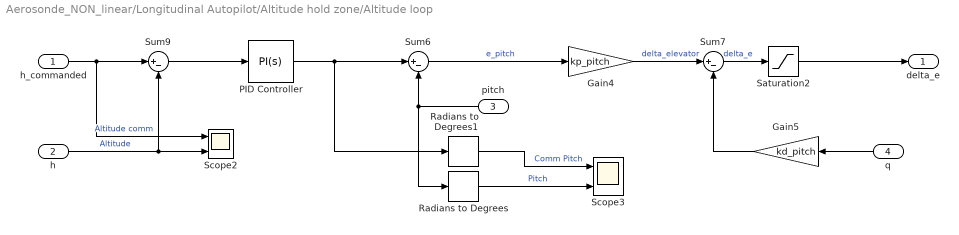
== system Aerosonde_NON_linear/Longitudinal Autopilot/Altitude hold zone/Altitude loop ==
  h_commanded : Inport
  h : Inport  Port=2
  pitch : Inport  Port=3
  q : Inport  Port=4
  Gain4 : Gain  Gain=kp_pitch
  Gain5 : Gain  Gain=kd_pitch
  PID Controller : slpidlib/PID Controller  Controller=PI  Form=Parallel  TimeDomain=Continuous-time  UseExternalTs=off  SampleTime=-1  IntegratorMethod=Forward Euler  FilterMethod=Forward Euler  ControllerParametersSource=internal  P=kp_h  I=ki_h  UseKiTs=off  D=0  N=100  UseFilter=on  TunerSelectOption=Transfer Function Based (PID Tuner App)  InitialConditionSource=internal  InitialConditionForIntegrator=0  InitialConditionForFilter=0  DifferentiatorICPrevScaledInput=0  ExternalReset=none  TrackingMode=off  Kt=1  LimitOutput=on  SatLimitsSource=internal  UpperSaturationLimit=deg2rad(20)  LowerSaturationLimit=deg2rad(-20)  LinearizeAsGain=on  AntiWindupMode=clamping  Kb=1  LimitIntegrator=off  UpperIntegratorSaturationLimit=inf  LowerIntegratorSaturationLimit=-inf  POutMin=[]  POutMax=[]  IOutMin=[]  IOutMax=[]  DOutMin=[]  DOutMax=[]  NOutMin=[]  NOutMax=[]  SumOutMin=[]  SumOutMax=[]  SaturationOutMin=[]  SaturationOutMax=[]  PParamMin=[]  PParamMax=[]  IParamMin=[]  IParamMax=[]  DParamMin=[]  DParamMax=[]  NParamMin=[]  NParamMax=[]  KbParamMin=[]  KbParamMax=[]  KtParamMin=[]  KtParamMax=[]  KbOutMin=[]  KbOutMax=[]  KtOutMin=[]  KtOutMax=[]  IntegratorOutMin=[]  IntegratorOutMax=[]  FilterOutMin=[]  FilterOutMax=[]  SumI1OutMin=[]  SumI1OutMax=[]  SumI2OutMin=[]  SumI2OutMax=[]  SumI3OutMin=[]  SumI3OutMax=[]  SumI4OutMin=[]  SumI4OutMax=[]  SumDOutMin=[]  SumDOutMax=[]  DifferentiatorOutMin=[]  DifferentiatorOutMax=[]  FilterDiffOutCoefMin=[]  FilterDiffOutCoefMax=[]  ReciprocalOutMin=[]  ReciprocalOutMax=[]  SumDenOutMin=[]  SumDenOutMax=[]  SumNumOutMin=[]  SumNumOutMax=[]  DivideOutMin=[]  DivideOutMax=[]  UdiffTsProdOutMin=[]  UdiffTsProdOutMax=[]  NTsProdOutMin=[]  NTsProdOutMax=[]  UintegralTsProdOutMin=[]  UintegralTsProdOutMax=[]  UngainTsProdOutMin=[]  UngainTsProdOutMax=[]  ClampingZeroOutDataTypeStr=Inherit: Inherit via back propagation  ClampingZeroOutMin=[]  ClampingZeroOutMax=[]  FilterDenConstantOutDataTypeStr=Inherit: Inherit via back propagation  FilterDenConstantOutMin=[]  FilterDenConstantOutMax=[]  PCopyOutDataTypeStr=Inherit: Inherit via back propagation  PCopyOutMin=[]  PCopyOutMax=[]  NCopyOutDataTypeStr=Inherit: Inherit via back propagation  NCopyOutMin=[]  NCopyOutMax=[]  IntegratorContinuousStateAttributes=''  IntegratorStateMustResolveToSignalObject=off  IntegratorRTWStateStorageClass=Auto  FilterContinuousStateAttributes=''  FilterStateMustResolveToSignalObject=off  FilterRTWStateStorageClass=Auto  ParallelPVariant=InternalParameters  IdealPVariant=Disabled  IVariant=InternalParameters  DVariant=Disabled  IntegratorVariant=Continuous  SatVariant=Enabled  AWVariant=ContClampingParallel  PCopyVariant=Disabled  TRVariant=Disabled  FdbkBlocksVariant=Forward  IdealPFdbkVariant=Disabled  SatFdbkVariant=Disabled  DerivativeFilterVariant=Disabled  NVariant=Disabled  NCopyVariant=Disabled_SignalSpec  FilterICVariant=Disabled  IntegratorICVariant=InternalICs  ExternalResetVariant=Disabled  TRSumVariant=Passthrough  SumFdbkVariant=Disabled  SumVariant=Sum_PI  TsampFilterVariant=InternalTs  TsampNgainVariant=Passthrough  TsampIntegralVariant=Disabled_SignalSpec  ExternalSaturationOutDataTypeStr=Inherit: Same as second input
  Radians to Degrees : simulink_extras/Transformations/Radians to Degrees
  Radians to Degrees1 : simulink_extras/Transformations/Radians to Degrees
  Saturation2 : Saturate  UpperLimit=0.43  LowerLimit=-0.43
  Scope2 : Scope  NumInputPorts=2
  Scope3 : Scope  NumInputPorts=2
  Sum6 : Sum  Inputs=|+-
  Sum7 : Sum  Inputs=|+-
  Sum9 : Sum  Inputs=|+-
  delta_e : Outport
  wires:
  Gain4/1 -> Sum7/1  "delta_elevator"
  PID Controller/1 -> Sum6/1, Radians to Degrees1/1
  Sum6/1 -> Gain4/1  "e_pitch"
  h/1 -> Scope2/2, Sum9/2  "Altitude"
  Sum9/1 -> PID Controller/1
  h_commanded/1 -> Scope2/1, Sum9/1  "Altitude comm"
  Sum7/1 -> Saturation2/1  "delta_e"
  pitch/1 -> Sum6/2, Radians to Degrees/1
  Saturation2/1 -> delta_e/1
  q/1 -> Gain5/1
  Gain5/1 -> Sum7/2
  Radians to Degrees/1 -> Scope3/2  "Pitch"
  Radians to Degrees1/1 -> Scope3/1  "Comm Pitch"

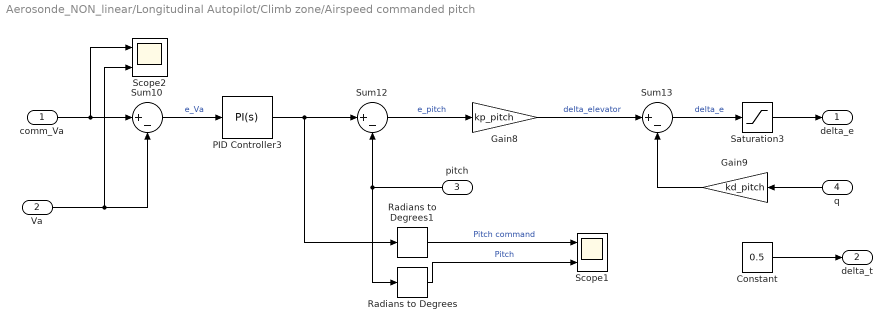
== system Aerosonde_NON_linear/Longitudinal Autopilot/Climb zone/Airspeed commanded pitch ==
  comm_Va : Inport
  Va : Inport  Port=2
  pitch : Inport  Port=3
  q : Inport  Port=4
  Constant : Constant  Value=0.5
  Gain8 : Gain  Gain=kp_pitch
  Gain9 : Gain  Gain=kd_pitch
  PID Controller3 : slpidlib/PID Controller  Controller=PI  Form=Parallel  TimeDomain=Continuous-time  UseExternalTs=off  SampleTime=-1  IntegratorMethod=Forward Euler  FilterMethod=Forward Euler  ControllerParametersSource=internal  P=kp_v2  I=ki_v2  UseKiTs=off  D=0  N=100  UseFilter=on  TunerSelectOption=Transfer Function Based (PID Tuner App)  InitialConditionSource=internal  InitialConditionForIntegrator=0  InitialConditionForFilter=0  DifferentiatorICPrevScaledInput=0  ExternalReset=none  TrackingMode=off  Kt=1  LimitOutput=on  SatLimitsSource=internal  UpperSaturationLimit=deg2rad(45)  LowerSaturationLimit=deg2rad(-20)  LinearizeAsGain=on  AntiWindupMode=clamping  Kb=1  LimitIntegrator=off  UpperIntegratorSaturationLimit=inf  LowerIntegratorSaturationLimit=-inf  POutMin=[]  POutMax=[]  IOutMin=[]  IOutMax=[]  DOutMin=[]  DOutMax=[]  NOutMin=[]  NOutMax=[]  SumOutMin=[]  SumOutMax=[]  SaturationOutMin=[]  SaturationOutMax=[]  PParamMin=[]  PParamMax=[]  IParamMin=[]  IParamMax=[]  DParamMin=[]  DParamMax=[]  NParamMin=[]  NParamMax=[]  KbParamMin=[]  KbParamMax=[]  KtParamMin=[]  KtParamMax=[]  KbOutMin=[]  KbOutMax=[]  KtOutMin=[]  KtOutMax=[]  IntegratorOutMin=[]  IntegratorOutMax=[]  FilterOutMin=[]  FilterOutMax=[]  SumI1OutMin=[]  SumI1OutMax=[]  SumI2OutMin=[]  SumI2OutMax=[]  SumI3OutMin=[]  SumI3OutMax=[]  SumI4OutMin=[]  SumI4OutMax=[]  SumDOutMin=[]  SumDOutMax=[]  DifferentiatorOutMin=[]  DifferentiatorOutMax=[]  FilterDiffOutCoefMin=[]  FilterDiffOutCoefMax=[]  ReciprocalOutMin=[]  ReciprocalOutMax=[]  SumDenOutMin=[]  SumDenOutMax=[]  SumNumOutMin=[]  SumNumOutMax=[]  DivideOutMin=[]  DivideOutMax=[]  UdiffTsProdOutMin=[]  UdiffTsProdOutMax=[]  NTsProdOutMin=[]  NTsProdOutMax=[]  UintegralTsProdOutMin=[]  UintegralTsProdOutMax=[]  UngainTsProdOutMin=[]  UngainTsProdOutMax=[]  ClampingZeroOutDataTypeStr=Inherit: Inherit via back propagation  ClampingZeroOutMin=[]  ClampingZeroOutMax=[]  FilterDenConstantOutDataTypeStr=Inherit: Inherit via back propagation  FilterDenConstantOutMin=[]  FilterDenConstantOutMax=[]  PCopyOutDataTypeStr=Inherit: Inherit via back propagation  PCopyOutMin=[]  PCopyOutMax=[]  NCopyOutDataTypeStr=Inherit: Inherit via back propagation  NCopyOutMin=[]  NCopyOutMax=[]  IntegratorContinuousStateAttributes=''  IntegratorStateMustResolveToSignalObject=off  IntegratorRTWStateStorageClass=Auto  FilterContinuousStateAttributes=''  FilterStateMustResolveToSignalObject=off  FilterRTWStateStorageClass=Auto  ParallelPVariant=InternalParameters  IdealPVariant=Disabled  IVariant=InternalParameters  DVariant=Disabled  IntegratorVariant=Continuous  SatVariant=Enabled  AWVariant=ContClampingParallel  PCopyVariant=Disabled  TRVariant=Disabled  FdbkBlocksVariant=Forward  IdealPFdbkVariant=Disabled  SatFdbkVariant=Disabled  DerivativeFilterVariant=Disabled  NVariant=Disabled  NCopyVariant=Disabled_SignalSpec  FilterICVariant=Disabled  IntegratorICVariant=InternalICs  ExternalResetVariant=Disabled  TRSumVariant=Passthrough  SumFdbkVariant=Disabled  SumVariant=Sum_PI  TsampFilterVariant=InternalTs  TsampNgainVariant=Passthrough  TsampIntegralVariant=Disabled_SignalSpec  ExternalSaturationOutDataTypeStr=Inherit: Same as second input
  Radians to Degrees : simulink_extras/Transformations/Radians to Degrees
  Radians to Degrees1 : simulink_extras/Transformations/Radians to Degrees
  Saturation3 : Saturate  UpperLimit=0.43  LowerLimit=-0.43
  Scope1 : Scope  NumInputPorts=2
  Scope2 : Scope  NumInputPorts=2
  Sum10 : Sum  Inputs=|+-
  Sum12 : Sum  Inputs=|+-
  Sum13 : Sum  Inputs=|+-
  delta_e : Outport
  delta_t : Outport  Port=2
  wires:
  Sum12/1 -> Gain8/1  "e_pitch"
  PID Controller3/1 -> Radians to Degrees1/1, Sum12/1
  Saturation3/1 -> delta_e/1
  Sum10/1 -> PID Controller3/1  "e_Va"
  Sum13/1 -> Saturation3/1  "delta_e"
  Gain8/1 -> Sum13/1  "delta_elevator"
  q/1 -> Gain9/1
  pitch/1 -> Radians to Degrees/1, Sum12/2
  comm_Va/1 -> Sum10/1, Scope2/1
  Va/1 -> Sum10/2, Scope2/2
  Gain9/1 -> Sum13/2
  Constant/1 -> delta_t/1
  Radians to Degrees/1 -> Scope1/2  "Pitch"
  Radians to Degrees1/1 -> Scope1/1  "Pitch command"

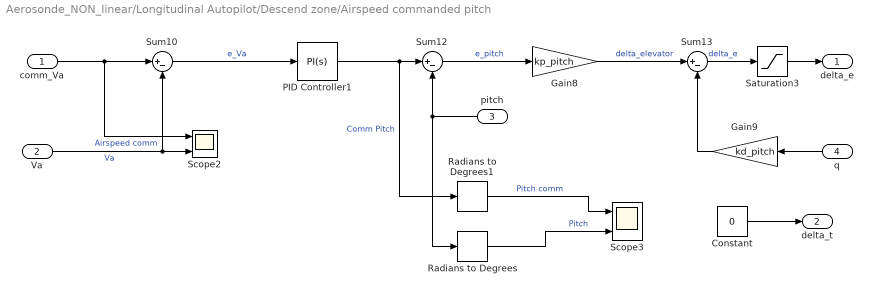
== system Aerosonde_NON_linear/Longitudinal Autopilot/Descend zone/Airspeed commanded pitch ==
  comm_Va : Inport
  Va : Inport  Port=2
  pitch : Inport  Port=3
  q : Inport  Port=4
  Constant : Constant  Value=0
  Gain8 : Gain  Gain=kp_pitch
  Gain9 : Gain  Gain=kd_pitch
  PID Controller1 : slpidlib/PID Controller  Controller=PI  Form=Parallel  TimeDomain=Continuous-time  UseExternalTs=off  SampleTime=-1  IntegratorMethod=Forward Euler  FilterMethod=Forward Euler  ControllerParametersSource=internal  P=kp_v2  I=ki_v2  UseKiTs=off  D=0  N=100  UseFilter=on  TunerSelectOption=Transfer Function Based (PID Tuner App)  InitialConditionSource=internal  InitialConditionForIntegrator=0  InitialConditionForFilter=0  DifferentiatorICPrevScaledInput=0  ExternalReset=none  TrackingMode=off  Kt=1  LimitOutput=on  SatLimitsSource=internal  UpperSaturationLimit=deg2rad(45)  LowerSaturationLimit=deg2rad(-20)  LinearizeAsGain=off  AntiWindupMode=clamping  Kb=1  LimitIntegrator=off  UpperIntegratorSaturationLimit=inf  LowerIntegratorSaturationLimit=-inf  POutMin=[]  POutMax=[]  IOutMin=[]  IOutMax=[]  DOutMin=[]  DOutMax=[]  NOutMin=[]  NOutMax=[]  SumOutMin=[]  SumOutMax=[]  SaturationOutMin=[]  SaturationOutMax=[]  PParamMin=[]  PParamMax=[]  IParamMin=[]  IParamMax=[]  DParamMin=[]  DParamMax=[]  NParamMin=[]  NParamMax=[]  KbParamMin=[]  KbParamMax=[]  KtParamMin=[]  KtParamMax=[]  KbOutMin=[]  KbOutMax=[]  KtOutMin=[]  KtOutMax=[]  IntegratorOutMin=[]  IntegratorOutMax=[]  FilterOutMin=[]  FilterOutMax=[]  SumI1OutMin=[]  SumI1OutMax=[]  SumI2OutMin=[]  SumI2OutMax=[]  SumI3OutMin=[]  SumI3OutMax=[]  SumI4OutMin=[]  SumI4OutMax=[]  SumDOutMin=[]  SumDOutMax=[]  DifferentiatorOutMin=[]  DifferentiatorOutMax=[]  FilterDiffOutCoefMin=[]  FilterDiffOutCoefMax=[]  ReciprocalOutMin=[]  ReciprocalOutMax=[]  SumDenOutMin=[]  SumDenOutMax=[]  SumNumOutMin=[]  SumNumOutMax=[]  DivideOutMin=[]  DivideOutMax=[]  UdiffTsProdOutMin=[]  UdiffTsProdOutMax=[]  NTsProdOutMin=[]  NTsProdOutMax=[]  UintegralTsProdOutMin=[]  UintegralTsProdOutMax=[]  UngainTsProdOutMin=[]  UngainTsProdOutMax=[]  ClampingZeroOutDataTypeStr=Inherit: Inherit via back propagation  ClampingZeroOutMin=[]  ClampingZeroOutMax=[]  FilterDenConstantOutDataTypeStr=Inherit: Inherit via back propagation  FilterDenConstantOutMin=[]  FilterDenConstantOutMax=[]  PCopyOutDataTypeStr=Inherit: Inherit via back propagation  PCopyOutMin=[]  PCopyOutMax=[]  NCopyOutDataTypeStr=Inherit: Inherit via back propagation  NCopyOutMin=[]  NCopyOutMax=[]  IntegratorContinuousStateAttributes=''  IntegratorStateMustResolveToSignalObject=off  IntegratorRTWStateStorageClass=Auto  FilterContinuousStateAttributes=''  FilterStateMustResolveToSignalObject=off  FilterRTWStateStorageClass=Auto  ParallelPVariant=InternalParameters  IdealPVariant=Disabled  IVariant=InternalParameters  DVariant=Disabled  IntegratorVariant=Continuous  SatVariant=Enabled  AWVariant=ContClampingParallel  PCopyVariant=Disabled  TRVariant=Disabled  FdbkBlocksVariant=Forward  IdealPFdbkVariant=Disabled  SatFdbkVariant=Disabled  DerivativeFilterVariant=Disabled  NVariant=Disabled  NCopyVariant=Disabled_SignalSpec  FilterICVariant=Disabled  IntegratorICVariant=InternalICs  ExternalResetVariant=Disabled  TRSumVariant=Passthrough  SumFdbkVariant=Disabled  SumVariant=Sum_PI  TsampFilterVariant=InternalTs  TsampNgainVariant=Passthrough  TsampIntegralVariant=Disabled_SignalSpec  ExternalSaturationOutDataTypeStr=Inherit: Same as second input
  Radians to Degrees : simulink_extras/Transformations/Radians to Degrees
  Radians to Degrees1 : simulink_extras/Transformations/Radians to Degrees
  Saturation3 : Saturate  UpperLimit=0.43  LowerLimit=-0.43
  Scope2 : Scope  NumInputPorts=2
  Scope3 : Scope  NumInputPorts=2
  Sum10 : Sum  Inputs=|+-
  Sum12 : Sum  Inputs=|+-
  Sum13 : Sum  Inputs=|+-
  delta_e : Outport
  delta_t : Outport  Port=2
  wires:
  Sum12/1 -> Gain8/1  "e_pitch"
  PID Controller1/1 -> Sum12/1, Radians to Degrees1/1  "Comm Pitch"
  Saturation3/1 -> delta_e/1
  Sum10/1 -> PID Controller1/1  "e_Va"
  Sum13/1 -> Saturation3/1  "delta_e"
  Gain8/1 -> Sum13/1  "delta_elevator"
  q/1 -> Gain9/1
  pitch/1 -> Radians to Degrees/1, Sum12/2
  comm_Va/1 -> Scope2/1, Sum10/1  "Airspeed comm"
  Va/1 -> Scope2/2, Sum10/2  "Va"
  Gain9/1 -> Sum13/2
  Constant/1 -> delta_t/1
  Radians to Degrees/1 -> Scope3/2  "Pitch"
  Radians to Degrees1/1 -> Scope3/1  "Pitch comm"

== matlab function Aerosonde_NON_linear/Longitudinal Autopilot/MATLAB Function2 ==
  data: h input; y output; h_comm input; delta_e input; delta_t input; num_case output
function [y,num_case] = switch_case_zone(h, h_comm, delta_e, delta_t)

%% Parameters

h_takeoff = 7;
h_hold = 10;
y = zeros(2,1);
num_case = 0;

%% Switch_case

switch h
    case h*(h<h_takeoff)
        num_case = 1;
        y(1)=delta_e(1);
        y(2)= delta_t(1);

    case h*(h>=h_takeoff && h<h_comm-h_hold)
        num_case = 2;
        y(1)=delta_e(2);
        y(2)= delta_t(2);

    case h*(h>=h_comm-h_hold && h<h_comm+h_hold)
        num_case = 3;
        y(1)=delta_e(3);
        y(2)= delta_t(3);
        
    case h*(h>=h_comm+h_hold)
        num_case = 4;
        y(1)=delta_e(4);
        y(2)= delta_t(4);

end

== matlab function Aerosonde_NON_linear/MATLAB Function ==
  data: x_dot output; x input; uu input
function x_dot  = aircraft_model_fcn(x,uu)

%% Definition Parameters
 gravity = 9.81; 
 mass = 13.5; %%kili
 Jx   = 0.8244; % Kg*m^2
 Jy   = 1.135;
 Jz   = 1.759;
 Jxz  = 0.1204;

 S=0.55; % m^2
 b=2.8956; % m
 c=0.18994; % m
 AR = b^2/S;

 S_prop = 0.2027; % m^2
 ro = 1.2682; % Kg/m^3
 k_motor = 80;
 k_t = 0;
 k_omega = 0;
%% Definitions of Gamma
 Gamma = Jx*Jz - Jxz^2;
 Gamma1 = Jxz*(Jx - Jy + Jz)/Gamma;
 Gamma2 = (Jz*(Jz - Jy) + Jxz^2)/Gamma;
 Gamma3 =Jz/Gamma;
 Gamma4 =Jxz/Gamma;
 Gamma5 =(Jz - Jx)/Jy;
 Gamma6 =Jxz/Jy;
 Gamma7 =((Jx - Jy)*Jx + Jxz^2)/Gamma;
 Gamma8 =Jx/Gamma;

%% Aerodynamic coefficient
% Longitudinal
 Cl_0 = 0.28;
 Cd_0 = 0.03;
 Cm_0 = -0.02338;
 Cl_alpha = 3.45;
 Cd_alpha = 0.3;
 Cm_alpha = -0.38;
 Cl_q = 0;
 Cd_q = 0;
 Cm_q = -3.6;
 Cl_delta_e=-0.36;
 Cd_delta_e= 0;
 Cm_delta_e= -0.5;
 C_prop = 1;
 M = 50;
 alpha_0 = 0.4712;
% epsilon = 0.1592;

% Lateral
 Cy_0 = 0;
 Cell_0 = 0;
 Cn_0 = 0;
 Cy_beta = -0.98;
 Cell_beta = -0.12;
 Cn_beta = 0.25;
 Cy_p= 0;
 Cell_p = -0.26;
 Cn_p = 0.022;
 Cy_r = 0;
 Cell_r = 0.14;
 Cn_r = -0.35;
 Cy_delta_a = 0;
 Cell_delta_a = 0.08;
 Cn_delta_a = 0.06;
 Cy_delta_r = -0.17;
 Cell_delta_r = 0.105;
 Cn_delta_r = -0.032;
 e=0.9;

% initial conditions
 pn0    = 0  % initial North position
 pe0    = 0 % initial East position
 pd0    = 0% initial Down position (negative altitude)
 u0     = 0.01  % initial velocity along body x-axis
 v0     =  0 % initial velocity along body y-axis
 w0     =  0 % initial velocity along body z-axis
 phi0   =  0 % initial roll angle
 theta0 =  0 % initial pitch angle
 psi0   =  0 % initial yaw angle
 p0     =  0 % initial body frame roll rate
 q0     =  0 % initial body frame pitch rate
 r0     =  0 % initial body frame yaw rate

X0 = [pn0; pe0; pd0; u0; v0; w0; phi0; theta0; psi0; p0; q0; r0];
%% State
    pn    = x(1);
    pe    = x(2);
    pd    = x(3);
    u     = x(4);
    v     = x(5);
    w     = x(6);
    phi   = x(7);
    theta = x(8);
    psi   = x(9);
    p     = x(10);
    q     = x(11);
    r     = x(12);

    delta_e = uu(1);
    delta_a = uu(2);
    delta_r = uu(3);
    delta_t = uu(4);
    Va = sqrt(u^2+v^2+w^2);
    alpha = atan2(w,u);
    beta  = asin(v);

%% Forces and Moments
sigma = (1+exp(-M*(alpha-alpha_0))+exp(M*(alpha+alpha_0)))/((1+exp(-M*(alpha-alpha_0)))*(1+exp(M*(alpha+alpha_0))));
Cl= (1-sigma)*(Cl_0+Cl_alpha*alpha)+sigma*(2*sign(alpha)*(sin(alpha))^2*cos(alpha));
Cd = Cd_0+(Cl_0+Cl_alpha*alpha)^2/(pi*e*AR);
Cx = -Cd*cos(alpha)+Cl*sin(alpha);
Cx_q = -Cd_q*cos(alpha)+Cl_q*sin(alpha);
Cx_delta_e=-Cd_delta_e*cos(alpha)+Cl_delta_e*sin(alpha);
Cz= -Cd*sin(alpha)-Cl*cos(alpha);
Cz_q = -Cd_q*sin(alpha) -Cl_q*cos(alpha);
Cz_delta_e = -Cd_delta_e*sin(alpha) - Cl_delta_e*cos(alpha);

fx = -mass*gravity*sin(theta) + 0.5*ro*Va^2*S*(Cx+Cx_q*c/(2*Va)*q+Cx_delta_e*delta_e) + 0.5*ro*S_prop*C_prop*((k_motor*delta_t)^2-Va^2);
fy = mass*gravity*cos(theta)*sin(phi) + 0.5*ro*Va^2*S*(Cy_0+Cy_beta*beta+Cy_p*b/(2*Va)*p+Cy_r*b/(2*Va)*r+Cy_delta_a*delta_a+Cy_delta_r*delta_r);
if(pd >= -0.25)
    fz = 0;
else
fz = mass*gravity*cos(theta)*cos(phi) + 0.5*ro*Va^2*S*(Cz+Cz_q*c/(2*Va)*q+Cz_delta_e*delta_e);
end
%[f_x; f_y; f_z] = [-P-mass*P.gravity*sin(theta); P.mass*P.gravity*cos(theta)*sin(phi); P.mass*P.gravity*cos(theta)*cos(phi)] + 0.5*ro*Va^2*S*[Cx+Cx_q*c/(2*Va)*q+Cx_delta_e*delta_e; Cy_0+Cy_beta*beta+Cy_p*b/(2*Va)*p+Cy_r*b/(2*Va)*r+Cy_delta_a*delta_a+Cy_delta_r*delta_r; Cz+Cz_q*c/(2*Va)*q+Cz_delta_e*delta_e]+0.5*ro*S_prop*C_prop*[(k_motor*delta_t)^2-Va^2; 0 ; 0];

ell = 0.5*ro*Va^2*S*(b*(Cell_0+Cell_beta*beta+Cell_p*b/(2*Va)*p+Cell_r*b/(2*Va)*r+Cell_delta_a*delta_a+Cell_delta_r*delta_r))-k_t*(k_omega*delta_t)^2;
if Va == 0
    m = 0;
    n =0;
else 
    m=0.5*ro*Va^2*S*(c*(Cm_0+Cm_alpha*alpha+Cm_q*c/(2*Va)*q+Cm_delta_e*delta_e)); 
    n= 0.5*ro*Va^2*S*(b*(Cn_0+Cn_beta*beta+Cn_p*b/(2*Va)*p+Cn_r*b/(2*Va)*r+Cn_delta_a*delta_a+Cn_delta_r*delta_r));
end
%[ell; m; n] = 0.5*ro*Va^2*S*[b*(Cell_0+Cell_beta*beta+Cell_p*b/(2*Va)*p+Cell_r*b/(2*Va)*r+Cell_delta_a*delta_a+Cell_delta_r*delta_r); c*(Cm_0+Cm_alpha*alpha+Cm_q*c/(2*Va)*q+Cm_delta_e*delta_e); b*(Cn_0+Cn_beta*beta+Cn_p*b/(2*Va)*p+Cn_r*b/(2*Va)*r+Cn_delta_a*delta_a+Cn_delta_r*delta_r)]+[-k_t*(k_omega*delta_t)^2; 0; 0];

%% Matrix 
R_b_to_v=[cos(theta)*cos(psi) sin(phi)*sin(theta)*cos(psi)-cos(phi)*sin(psi) cos(phi)*sin(theta)*cos(psi)+sin(phi)*sin(psi); cos(theta)*sin(psi) sin(phi)*sin(theta)*sin(psi)+cos(phi)*cos(psi) cos(phi)*sin(theta)*sin(psi)-sin(phi)*cos(psi); -sin(theta) sin(phi)*cos(theta) cos(psi)*cos(theta)];

%% Update State
% [pndot; pedot; pddot] = R_b_to_v * [u; v; w];
pndot = [cos(theta)*cos(psi) sin(phi)*sin(theta)*cos(psi)-cos(phi)*sin(psi) cos(phi)*sin(theta)*cos(psi)+sin(phi)*sin(psi)] * [u;v;w];
pedot = [cos(theta)*sin(psi) sin(phi)*sin(theta)*sin(psi)+cos(phi)*cos(psi) cos(phi)*sin(theta)*sin(psi)-sin(phi)*cos(psi)] * [u;v;w];
pddot = [-sin(theta) sin(phi)*cos(theta) cos(psi)*cos(theta)]* [u;v;w];

% [udot; vdot; wdot] = [r*v - q*w; p*w - r*u; q*u - p*v] + 1/m * [f_x; f_y; f_z];
udot = (r*v - q*w) + 1/mass * fx;
vdot = (p*w - r*u) + 1/mass * fy;
wdot = (q*u - p*v) + 1/mass * fz;

%[phidot; thetadot; psidot] = [1 sin(phi)*tan(theta) cos(phi)*tan(theta); 0 cos(phi) -sin(phi); 0 sin(phi)/cos(theta) cos(phi)/cos(theta)]*[p; q; r];
phidot = [1 sin(phi)*tan(theta) cos(phi)*tan(theta)]*[p; q; r];
thetadot =  [0 cos(phi) -sin(phi)]*[p; q; r];
psidot = [0 sin(phi)/cos(theta) cos(phi)/cos(theta)]*[p; q; r];

%[pdot; qdot; rdot] = [Gamma1*p*q-Gamma2*q*r; Gamma5*p*r-Gamma6*(p^2-r^2); Gamma7*p*q-Gamma1*q*r] + [Gamma3*ell+Gamma4*n; m/P.Jy; Gamma4*ell+Gamma8*n];
pdot = Gamma1*p*q-Gamma2*q*r+Gamma3*ell+Gamma4*n;
qdot = Gamma5*p*r-Gamma6*(p^2-r^2) + m/Jy;
rdot = Gamma7*p*q-Gamma1*q*r + Gamma4*ell+Gamma8*n;

sys = [pndot; pedot; pddot; udot; vdot; wdot; phidot; thetadot; psidot; pdot; qdot; rdot];
x_dot = sys';

== matlab function Aerosonde_NON_linear/MATLAB Function1 ==
  data: attitude input; u_ws output; v_ws output; w_ws output
function [ u_ws, v_ws, w_ws] = wind_fcn(attitude)

%% Wind model
    %% Input
    phi = attitude(1);
    theta = attitude(2);
    psi = attitude(3);
    %% Steady wind in NED frame
    wn_s = +0.5; %m/s
    we_s = 0.2; %m/s
    wd_s = 0.1; %m/s
    %% Steady wind in body frame
    u_ws = [cos(theta)*cos(psi) sin(phi)*sin(theta)*cos(psi)-cos(phi)*sin(psi) cos(phi)*sin(theta)*cos(psi)+sin(phi)*sin(psi)] * [wn_s;we_s;wd_s];
    v_ws = [cos(theta)*sin(psi) sin(phi)*sin(theta)*sin(psi)+cos(phi)*cos(psi) cos(phi)*sin(theta)*sin(psi)-sin(phi)*cos(psi)] * [wn_s;we_s;wd_s];
    w_ws = [-sin(theta) sin(phi)*cos(theta) cos(psi)*cos(theta)]* [wn_s;we_s;wd_s];
